simulink model "smoczek"  (R2022a)
settings: Solver=FixedStepAuto  StartTime=0.0  StopTime=100  FixedStep=0.25  RelTol=1e-7
values from neighbouring files (symbols this model uses):
  m = 10    [T.mat]    (also in x.mat)
  T = [1 1 1 1.5 1 2 1 2.5 1 3 1 3.5 ... (722 elements, 2x361)]    [T.mat]    (also in untitled2.m = T'; x.mat)
settings Model: Creator=sucho  LastModifiedBy=sucho

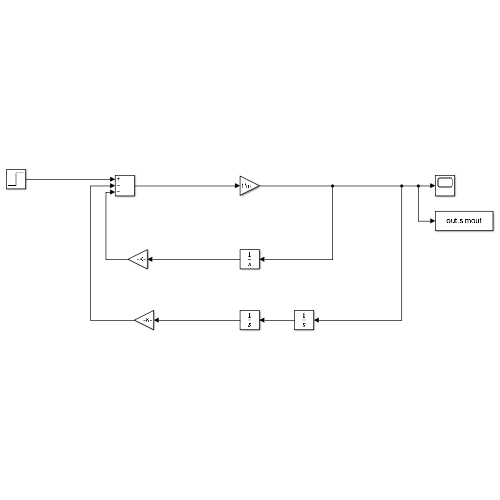
[thumbnail: Simulink's stored preview of the top-level diagram]
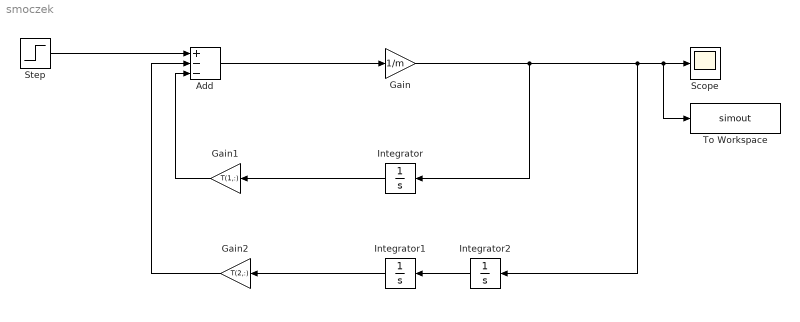
== system smoczek ==
  Add : Sum  Inputs=+--
  Gain : Gain  Gain=1/m
  Gain1 : Gain  Gain=T(1,:)
  Gain2 : Gain  Gain=T(2,:)
  Integrator : Integrator
  Integrator1 : Integrator
  Integrator2 : Integrator
  Scope : Scope
  Step : Step  Time=0  SampleTime=0
  To Workspace : ToWorkspace  VariableName=simout  SaveFormat=Timeseries  SampleTime=-1
  wires:
  Step/1 -> Add/1
  Add/1 -> Gain/1
  Gain/1 -> Integrator/1, Integrator2/1, To Workspace/1, Scope/1
  Integrator/1 -> Gain1/1
  Integrator1/1 -> Gain2/1
  Integrator2/1 -> Integrator1/1
  Gain1/1 -> Add/3
  Gain2/1 -> Add/2
